simulink model "simulate_fuzzy"  (R2014b)
settings: Solver=ode4  StartTime=0.0  StopTime=20.0  FixedStep=0.01  RelTol=1e-3
undefined symbols (not defined in the file or in its folder): test
libraries: fuzblock x1
settings Model: Creator=nk  LastModifiedBy=nk

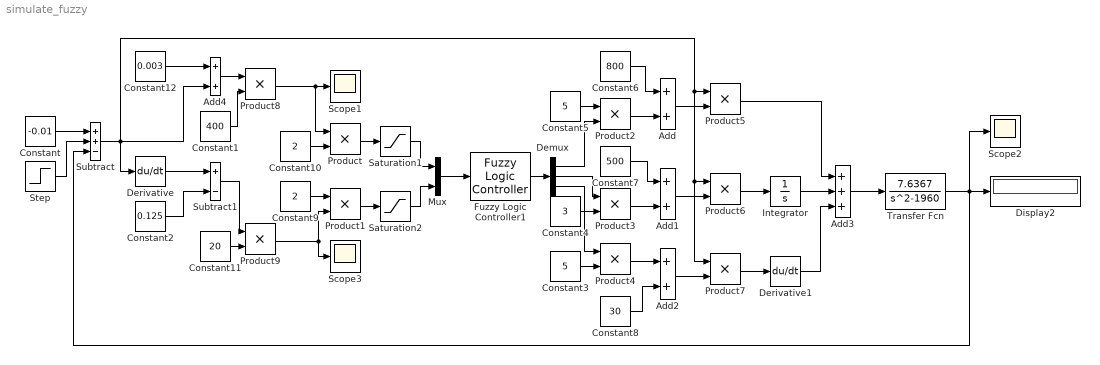
== system simulate_fuzzy ==
  Add{,1..2,4} (4 alike) : Sum
  Add3 : Sum  Inputs=+++
  Constant : Constant  Value=-0.01
  Constant1 : Constant  Value=400
  Constant10 : Constant  Value=2
  Constant11 : Constant  Value=20
  Constant12 : Constant  Value=0.003
  Constant2 : Constant  Value=0.125
  Constant3 : Constant  Value=5
  Constant4 : Constant  Value=3
  Constant5 : Constant  Value=5
  Constant6 : Constant  Value=800
  Constant7 : Constant  Value=500
  Constant8 : Constant  Value=30
  Constant9 : Constant  Value=2
  Demux : Demux  Outputs=3
  Derivative : Derivative
  Derivative1 : Derivative
  Display2 : Display
  Fuzzy Logic Controller1 : fuzblock/Fuzzy Logic  Controller  fis=[test]
  Integrator : Integrator
  Mux : Mux  Inputs=2
  Product{,1..9} (10 alike) : Product
  Saturation1 : Saturate
  Saturation2 : Saturate
  Scope1 : Scope
      settings: YMin=-0.012  YMax=-0.007
  Scope2 : Scope
      settings: YMin=-0.012  YMax=-0.007  SaveName=ScopeData2
  Scope3 : Scope
      settings: TimeRange=1.368821292775666  YMin=-0.007921875000000002  YMax=-0.007546875000000002
  Step : Step  Time=10  After=0.001  SampleTime=0
  Subtract : Sum  Inputs=++-
  Subtract1 : Sum  Inputs=+-
  Transfer Fcn : TransferFcn  Numerator=[7.6367]  Denominator=[1 0 -1960]
  wires:
  Subtract/1 -> Product5/1, Product7/1, Product6/1, Add4/2, Derivative/1
  Mux/1 -> Fuzzy Logic Controller1/1
  Fuzzy Logic Controller1/1 -> Demux/1
  Demux/1 -> Product2/2
  Demux/2 -> Product3/1
  Demux/3 -> Product4/1
  Constant5/1 -> Product2/1
  Constant4/1 -> Product3/2
  Constant3/1 -> Product4/2
  Product2/1 -> Add/2
  Constant6/1 -> Add/1
  Product3/1 -> Add1/2
  Constant7/1 -> Add1/1
  Product4/1 -> Add2/1
  Constant8/1 -> Add2/2
  Add/1 -> Product5/2
  Add1/1 -> Product6/2
  Add2/1 -> Product7/2
  Product7/1 -> Derivative1/1
  Product6/1 -> Integrator/1
  Product5/1 -> Add3/1
  Integrator/1 -> Add3/2
  Derivative1/1 -> Add3/3
  Add3/1 -> Transfer Fcn/1
  Transfer Fcn/1 -> Display2/1, Subtract/3, Scope2/1
  Step/1 -> Subtract/2
  Constant/1 -> Subtract/1
  Saturation2/1 -> Mux/2
  Saturation1/1 -> Mux/1
  Product/1 -> Saturation1/1
  Product1/1 -> Saturation2/1
  Constant9/1 -> Product1/1
  Constant10/1 -> Product/2
  Product9/1 -> Product1/2, Scope3/1
  Product8/1 -> Product/1, Scope1/1
  Constant11/1 -> Product9/2
  Constant2/1 -> Subtract1/2
  Derivative/1 -> Subtract1/1
  Subtract1/1 -> Product9/1
  Add4/1 -> Product8/1
  Constant1/1 -> Product8/2
  Constant12/1 -> Add4/1
